simulink model "Practica_2"  (R2024b)
settings: Solver=VariableStepAuto  StartTime=0.0  StopTime=10  RelTol=1e-3
InitFcn:
  | Ip = 0.0079;     % kg*m^2  (Momento de inercia del péndulo)
  | Mc = 0.7031;     % kg      (Masa del carro)
  | lp = 0.3302;     % m       (Distancia al centro de gravedad)
  | Mp = 0.23;       % kg      (Masa del péndulo)
  | Fc = 0;          % N       (Fuerza aplicada al carro)
  | Beq = 4.3;       % Ns/m    (Coeficiente de amortiguamiento equivalente)
  | g = 9.81;        % m/s^2   (Gravedad)
  | Bp = 0.0024;     % Nms/rad (Coeficiente de amortiguamiento en el péndulo)
settings Model: Creator=RAM  LastModifiedBy=RAM

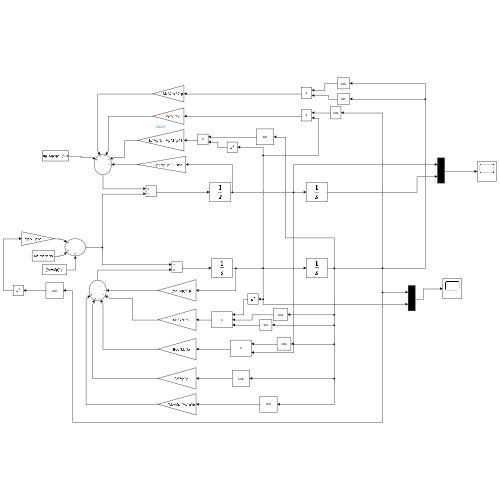
[thumbnail: Simulink's stored preview of the top-level diagram]
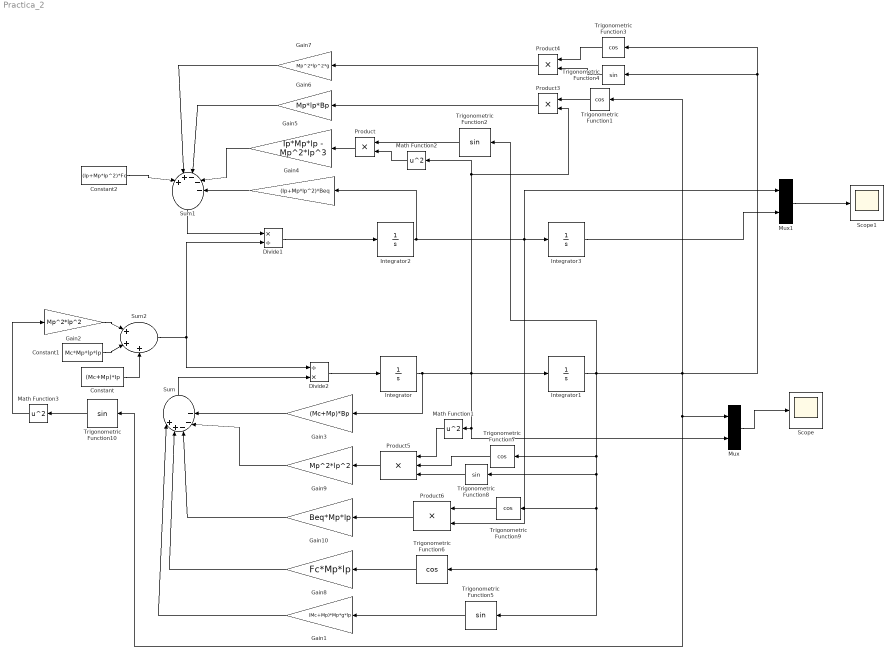
== system Practica_2 ==
  Constant : Constant  Value=(Mc+Mp)*Ip
  Constant1 : Constant  Value=Mc*Mp*lp*lp
  Constant2 : Constant  Value=(Ip+Mp*lp^2)*Fc
  Divide1 : Product  Inputs=*/
  Divide2 : Product  Inputs=/*
  Gain1 : Gain  Gain=(Mc+Mp)*Mp*g*lp
  Gain10 : Gain  Gain=Beq*Mp*lp
  Gain2 : Gain  Gain=Mp^2*lp^2
  Gain3 : Gain  Gain=(Mc+Mp)*Bp
  Gain4 : Gain  Gain=(Ip+Mp*lp^2)*Beq
  Gain5 : Gain  Gain=Ip*Mp*lp - Mp^2*lp^3
  Gain6 : Gain  Gain=Mp*lp*Bp
  Gain7 : Gain  Gain=Mp^2*lp^2*g
  Gain8 : Gain  Gain=Fc*Mp*lp
  Gain9 : Gain  Gain=Mp^2*lp^2
  Integrator : Integrator
  Integrator1 : Integrator  InitialCondition=1 * pi/180
  Integrator2 : Integrator
  Integrator3 : Integrator
  Math Function1 : Math  Operator=square
  Math Function2 : Math  Operator=square
  Math Function3 : Math  Operator=square
  Mux : Mux  Inputs=2
  Mux1 : Mux  Inputs=2
  Product{,3..4,6} (4 alike) : Product
  Product5 : Product  Inputs=3
  Scope : Scope
  Scope1 : Scope
  Sum : Sum  Inputs=|++---
  Sum1 : Sum  Inputs=|++---
  Sum2 : Sum  Inputs=|+++
  Trigonometric Function{1,3,6..7,9} (5 alike) : Trigonometry  Operator=cos
  Trigonometric Function{2,4..5,8,10} (5 alike) : Trigonometry
  wires:
  Mux1/1 -> Scope1/1
  Product6/1 -> Gain10/1
  Integrator2/1 -> Gain4/1, Mux1/1, Integrator3/1, Product6/2
  Trigonometric Function10/1 -> Math Function3/1
  Constant2/1 -> Sum1/1
  Sum2/1 -> Divide1/2, Divide2/1
  Product/1 -> Gain5/1
  Divide2/1 -> Integrator/1
  Constant/1 -> Sum2/3
  Gain10/1 -> Sum/3
  Product3/1 -> Gain6/1
  Mux/1 -> Scope/1
  Gain1/1 -> Sum/1
  Gain3/1 -> Sum/5
  Gain2/1 -> Sum2/1
  Trigonometric Function7/1 -> Product5/2
  Trigonometric Function3/1 -> Product4/1
  Gain7/1 -> Sum1/2
  Trigonometric Function1/1 -> Product3/1
  Integrator/1 -> Mux/2, Math Function1/1, Integrator1/1, Product3/2, Math Function2/1, Gain3/1
  Trigonometric Function4/1 -> Product4/2
  Divide1/1 -> Integrator2/1
  Integrator3/1 -> Mux1/2
  Sum1/1 -> Divide1/1
  Math Function3/1 -> Gain2/1
  Gain8/1 -> Sum/2
  Gain9/1 -> Sum/4
  Constant1/1 -> Sum2/2
  Integrator1/1 -> Trigonometric Function10/1, Mux/1, Trigonometric Function3/1, Trigonometric Function4/1, Trigonometric Function1/1, Trigonometric Function2/1, Trigonometric Function7/1, Trigonometric Function8/1, Trigonometric Function9/1, Trigonometric Function6/1, Trigonometric Function5/1
  Gain4/1 -> Sum1/5
  Trigonometric Function9/1 -> Product6/1
  Trigonometric Function5/1 -> Gain1/1
  Trigonometric Function6/1 -> Gain8/1
  Trigonometric Function2/1 -> Product/1
  Product4/1 -> Gain7/1
  Product5/1 -> Gain9/1
  Gain5/1 -> Sum1/4
  Gain6/1 -> Sum1/3
  Trigonometric Function8/1 -> Product5/3
  Math Function1/1 -> Product5/1
  Math Function2/1 -> Product/2
  Sum/1 -> Divide2/2
